simulink model "Quanser_Posicion_fuzzy"  (R2016a)
settings: Solver=VariableStepAuto  StartTime=0.0  StopTime=3000  RelTol=1e-3
undefined symbols (not defined in the file or in its folder): QuanserPositionFuzzy
libraries: fuzblock x1
settings Model: Creator=Daniel  LastModifiedBy=Daniel

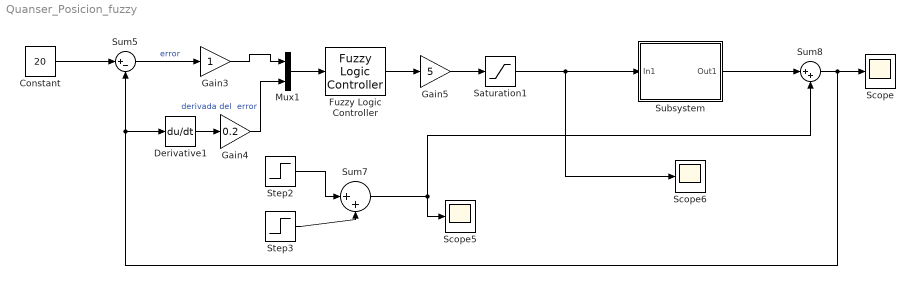
== system Quanser_Posicion_fuzzy ==
  Constant : Constant  Value=20
  Derivative1 : Derivative
  Fuzzy Logic Controller : fuzblock/Fuzzy Logic  Controller  fis=[QuanserPositionFuzzy]
  Gain3 : Gain
  Gain4 : Gain  Gain=0.2
  Gain5 : Gain  Gain=5
  Mux1 : Mux  Inputs=2
  Saturation1 : Saturate  UpperLimit=0.1  LowerLimit=-0.1
  Scope : Scope
  Scope5 : Scope
  Scope6 : Scope
  Step2 : Step  Time=4  After=0.2  SampleTime=0
  Step3 : Step  Time=5  After=-0.2  SampleTime=0
  Subsystem : Subsystem
  Sum5 : Sum  Inputs=|+-
  Sum7 : Sum  Inputs=|++
  Sum8 : Sum  Inputs=|++
  wires:
  Sum5/1 -> Gain3/1  "error"
  Gain3/1 -> Mux1/1
  Gain5/1 -> Saturation1/1
  Derivative1/1 -> Gain4/1
  Gain4/1 -> Mux1/2  "derivada del  error"
  Saturation1/1 -> Subsystem/1(In1), Scope6/1
  Step2/1 -> Sum7/1
  Step3/1 -> Sum7/2
  Sum7/1 -> Scope5/1, Sum8/2
  Sum8/1 -> Scope/1, Derivative1/1, Sum5/2
  Constant/1 -> Sum5/1
  Subsystem/1(Out1) -> Sum8/1
  Mux1/1 -> Fuzzy Logic Controller/1
  Fuzzy Logic Controller/1 -> Gain5/1

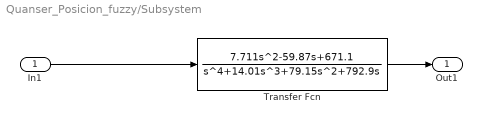
== system Quanser_Posicion_fuzzy/Subsystem ==
  In1 : Inport
  Transfer Fcn : TransferFcn  Numerator=[7.711 -59.87 671.1]  Denominator=[1 14.01 79.15 792.9 0]
  Out1 : Outport
  wires:
  Transfer Fcn/1 -> Out1/1
  In1/1 -> Transfer Fcn/1
